simulink subsystem "Torque_vectoring_old"  (R2022a)
settings: Solver=VariableStepAuto  StartTime=0.0  StopTime=10.0  RelTol=1e-3
undefined symbols (not defined in the file): pac, param_vdc
libraries: slpidlib x1
settings Model: Creator=jutri  LastModifiedBy=Usuario
settings ModelReferenceCC: EnableRefExpFcnMdlSchedulingChecks=off
settings RTWCC: Description=Generic Real-Time Target  GPUComputeCapability=5.0

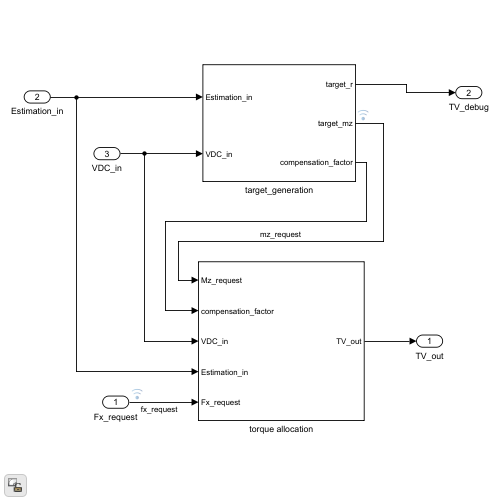
[thumbnail: Simulink's stored preview of the top-level diagram]
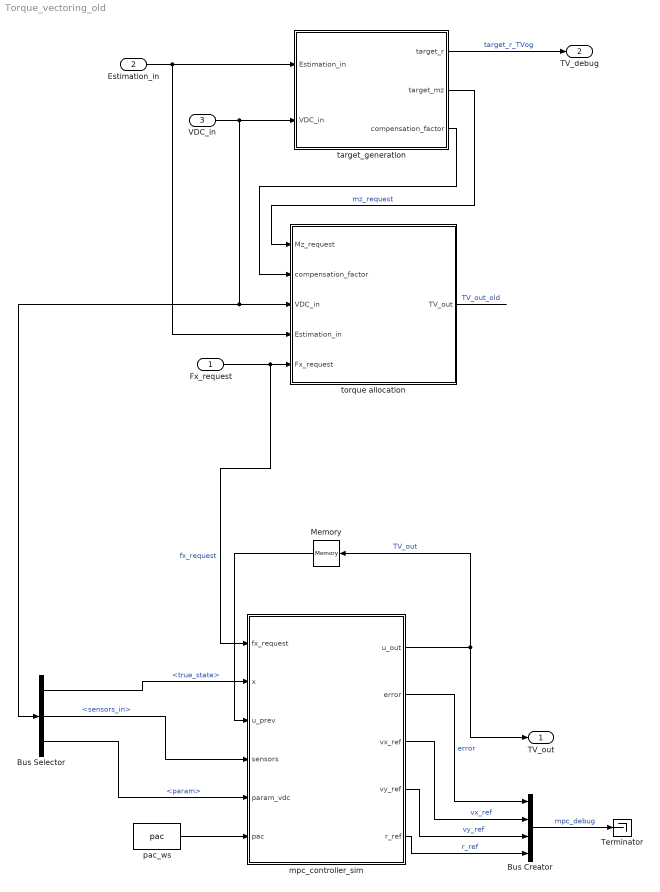
== system Torque_vectoring_old ==
  Fx_request : Inport
  Estimation_in : Inport  Port=2
  VDC_in : Inport  Port=3
  Bus Creator : BusCreator  Inputs=4
  Bus Selector : BusSelector  OutputSignals=true_state,sensors_in,param
  Memory : Memory  InitialCondition=[0;0;0;0]
  Terminator : Terminator
  mpc_controller_sim : MATLAB Function  TreatAsAtomicUnit=on
  pac_ws : Constant  Value=pac  OutDataTypeStr=Bus: pacBus
  target_generation : Subsystem
  torque allocation : Subsystem
  TV_out : Outport
  TV_debug : Outport  Port=2
  wires:
  Fx_request/1 -> torque allocation/5(Fx_request), mpc_controller_sim/1(fx_request)  "fx_request"
  torque allocation/1(TV_out) -> ?  "TV_out_old"
  target_generation/1(target_r) -> TV_debug/1  "target_r_TVog"
  Estimation_in/1 -> torque allocation/4(Estimation_in), target_generation/1(Estimation_in)
  VDC_in/1 -> Bus Selector/1, torque allocation/3(VDC_in), target_generation/2(VDC_in)
  target_generation/2(target_mz) -> torque allocation/1(Mz_request)  "mz_request"
  target_generation/3(compensation_factor) -> torque allocation/2(compensation_factor)
  mpc_controller_sim/1(u_out) -> Memory/1, TV_out/1  "TV_out"
  Memory/1 -> mpc_controller_sim/3(u_prev)
  Bus Selector/3 -> mpc_controller_sim/5(param_vdc)  "<param>"
  Bus Selector/2 -> mpc_controller_sim/4(sensors)  "<sensors_in>"
  Bus Selector/1 -> mpc_controller_sim/2(x)  "<true_state>"
  pac_ws/1 -> mpc_controller_sim/6(pac)
  mpc_controller_sim/2(error) -> Bus Creator/1  "error"
  Bus Creator/1 -> Terminator/1  "mpc_debug"
  mpc_controller_sim/3(vx_ref) -> Bus Creator/2  "vx_ref"
  mpc_controller_sim/4(vy_ref) -> Bus Creator/3  "vy_ref"
  mpc_controller_sim/5(r_ref) -> Bus Creator/4  "r_ref"

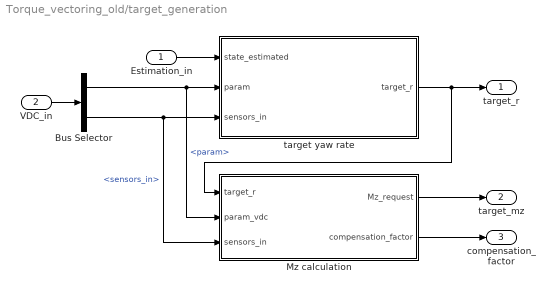
== system Torque_vectoring_old/target_generation ==
  Estimation_in : Inport
  VDC_in : Inport  Port=2
  Bus Selector : BusSelector  OutputSignals=param,sensors_in
  Mz calculation : Subsystem
  target yaw rate : Subsystem
  target_r : Outport
  target_mz : Outport  Port=2
  compensation_factor : Outport  Port=3
  wires:
  Mz calculation/2(compensation_factor) -> compensation_factor/1
  Bus Selector/2 -> target yaw rate/3(sensors_in), Mz calculation/3(sensors_in)  "<sensors_in>"
  Bus Selector/1 -> target yaw rate/2(param), Mz calculation/2(param_vdc)  "<param>"
  Estimation_in/1 -> target yaw rate/1(state_estimated)
  target yaw rate/1(target_r) -> target_r/1, Mz calculation/1(target_r)
  Mz calculation/1(Mz_request) -> target_mz/1
  VDC_in/1 -> Bus Selector/1

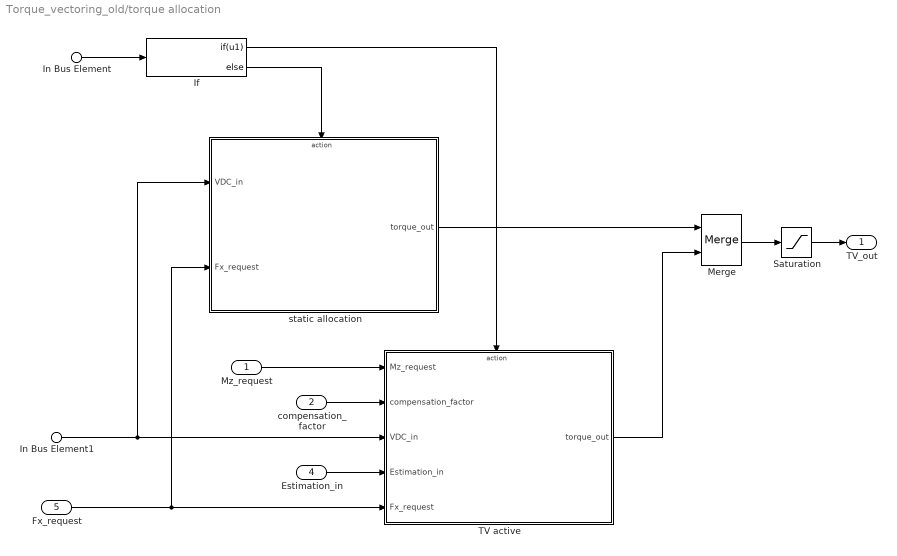
== system Torque_vectoring_old/torque allocation ==
  Mz_request : Inport
  compensation_factor : Inport  Port=2
  In Bus Element1 : Inport  Port=3  PortName=VDC_in
  In Bus Element : Inport  Port=3  PortName=VDC_in  Element=param.TV_active
  Estimation_in : Inport  Port=4
  Fx_request : Inport  Port=5
  If : If  IfExpression=u1
  Merge : Merge
  Saturation : Saturate  UpperLimit=param_vdc.torque_limit_positive  LowerLimit=param_vdc.torque_limit_negative
  TV active : Subsystem  TreatAsAtomicUnit=on
  static allocation : Subsystem  TreatAsAtomicUnit=on
  TV_out : Outport
  wires:
  compensation_factor/1 -> TV active/2(compensation_factor)
  Saturation/1 -> TV_out/1
  In Bus Element/1 -> If/1
  If/2 -> static allocation/Action
  If/1 -> TV active/Action
  Merge/1 -> Saturation/1
  TV active/1(torque_out) -> Merge/2
  static allocation/1(torque_out) -> Merge/1
  In Bus Element1/1 -> TV active/3(VDC_in), static allocation/1(VDC_in)
  Fx_request/1 -> TV active/5(Fx_request), static allocation/2(Fx_request)
  Estimation_in/1 -> TV active/4(Estimation_in)
  Mz_request/1 -> TV active/1(Mz_request)

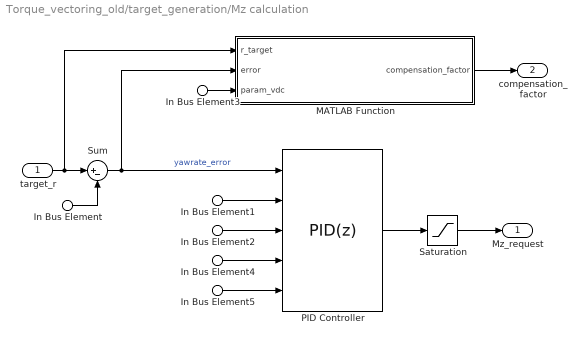
== system Torque_vectoring_old/target_generation/Mz calculation ==
  target_r : Inport
  In Bus Element3 : Inport  Port=2  PortName=param_vdc
  In Bus Element1 : Inport  Port=2  PortName=param_vdc  Element=TV_Kp
  In Bus Element2 : Inport  Port=2  PortName=param_vdc  Element=TV_Ki
  In Bus Element4 : Inport  Port=2  PortName=param_vdc  Element=TV_Kd
  In Bus Element5 : Inport  Port=2  PortName=param_vdc  Element=TV_N
  In Bus Element : Inport  Port=3  PortName=sensors_in  Element=IMU.r
  MATLAB Function : MATLAB Function  TreatAsAtomicUnit=on
  PID Controller : slpidlib/PID Controller  Controller=PID  Form=Parallel  TimeDomain=Discrete-time  UseExternalTs=off  SampleTime=-1  IntegratorMethod=Forward Euler  FilterMethod=Forward Euler  ControllerParametersSource=external  P=1  I=1  UseKiTs=off  D=0  N=100  UseFilter=on  TunerSelectOption=Transfer Function Based (PID Tuner App)  InitialConditionSource=internal  InitialConditionForIntegrator=0  InitialConditionForFilter=0  DifferentiatorICPrevScaledInput=0  ExternalReset=none  TrackingMode=off  Kt=1  LimitOutput=off  SatLimitsSource=internal  UpperSaturationLimit=inf  LowerSaturationLimit=-inf  LinearizeAsGain=on  AntiWindupMode=none  Kb=1  POutMin=[]  POutMax=[]  IOutMin=[]  IOutMax=[]  DOutMin=[]  DOutMax=[]  NOutMin=[]  NOutMax=[]  SumOutMin=[]  SumOutMax=[]  SaturationOutMin=[]  SaturationOutMax=[]  PParamMin=[]  PParamMax=[]  IParamMin=[]  IParamMax=[]  DParamMin=[]  DParamMax=[]  NParamMin=[]  NParamMax=[]  KbParamMin=[]  KbParamMax=[]  KtParamMin=[]  KtParamMax=[]  KbOutMin=[]  KbOutMax=[]  KtOutMin=[]  KtOutMax=[]  IntegratorOutMin=[]  IntegratorOutMax=[]  FilterOutMin=[]  FilterOutMax=[]  SumI1OutMin=[]  SumI1OutMax=[]  SumI2OutMin=[]  SumI2OutMax=[]  SumI3OutMin=[]  SumI3OutMax=[]  SumI4OutMin=[]  SumI4OutMax=[]  SumDOutMin=[]  SumDOutMax=[]  DifferentiatorOutMin=[]  DifferentiatorOutMax=[]  FilterDiffOutCoefMin=[]  FilterDiffOutCoefMax=[]  ReciprocalOutMin=[]  ReciprocalOutMax=[]  SumDenOutMin=[]  SumDenOutMax=[]  SumNumOutMin=[]  SumNumOutMax=[]  DivideOutMin=[]  DivideOutMax=[]  UdiffTsProdOutMin=[]  UdiffTsProdOutMax=[]  NTsProdOutMin=[]  NTsProdOutMax=[]  UintegralTsProdOutMin=[]  UintegralTsProdOutMax=[]  UngainTsProdOutMin=[]  UngainTsProdOutMax=[]  ClampingZeroOutDataTypeStr=Inherit: Inherit via back propagation  ClampingZeroOutMin=[]  ClampingZeroOutMax=[]  FilterDenConstantOutDataTypeStr=Inherit: Inherit via back propagation  FilterDenConstantOutMin=[]  FilterDenConstantOutMax=[]  PCopyOutDataTypeStr=Inherit: Inherit via back propagation  PCopyOutMin=[]  PCopyOutMax=[]  NCopyOutDataTypeStr=Inherit: Inherit via back propagation  NCopyOutMin=[]  NCopyOutMax=[]  IntegratorContinuousStateAttributes=''  IntegratorStateMustResolveToSignalObject=off  IntegratorRTWStateStorageClass=Auto  FilterContinuousStateAttributes=''  FilterStateMustResolveToSignalObject=off  FilterRTWStateStorageClass=Auto  ParallelPVariant=ExternalParameters  IdealPVariant=Disabled  IVariant=ExternalParameters  DVariant=ExternalParameters  IntegratorVariant=Discrete  SatVariant=Disabled  AWVariant=Passthrough  PCopyVariant=Disabled  TRVariant=Disabled  FdbkBlocksVariant=Forward  IdealPFdbkVariant=Disabled  SatFdbkVariant=Disabled  DerivativeFilterVariant=ForwardEulerFilter  NVariant=ExternalParameters  NCopyVariant=Disabled  FilterICVariant=InternalICsFilter  IntegratorICVariant=InternalICs  ExternalResetVariant=Disabled  TRSumVariant=Passthrough  SumFdbkVariant=Disabled  SumVariant=Sum_PID  TsampFilterVariant=InternalTs  TsampNgainVariant=Passthrough  TsampIntegralVariant=Passthrough  ExternalSaturationOutDataTypeStr=Inherit: Same as second input  aMode=0
  Saturation : Saturate  UpperLimit=param_vdc.max_mz  LowerLimit=-param_vdc.max_mz
  Sum : Sum  Inputs=|+-
  Mz_request : Outport
  compensation_factor : Outport  Port=2
  wires:
  MATLAB Function/1(compensation_factor) -> compensation_factor/1
  In Bus Element5/1 -> PID Controller/5
  In Bus Element4/1 -> PID Controller/4
  In Bus Element2/1 -> PID Controller/3
  In Bus Element1/1 -> PID Controller/2
  In Bus Element3/1 -> MATLAB Function/3(param_vdc)
  Sum/1 -> PID Controller/1, MATLAB Function/2(error)  "yawrate_error"
  In Bus Element/1 -> Sum/2
  target_r/1 -> Sum/1, MATLAB Function/1(r_target)
  PID Controller/1 -> Saturation/1
  Saturation/1 -> Mz_request/1

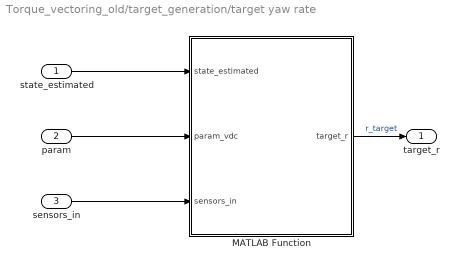
== system Torque_vectoring_old/target_generation/target yaw rate ==
  state_estimated : Inport
  param : Inport  Port=2
  sensors_in : Inport  Port=3
  MATLAB Function : MATLAB Function  TreatAsAtomicUnit=on
  target_r : Outport
  wires:
  MATLAB Function/1(target_r) -> target_r/1  "r_target"
  sensors_in/1 -> MATLAB Function/3(sensors_in)
  param/1 -> MATLAB Function/2(param_vdc)
  state_estimated/1 -> MATLAB Function/1(state_estimated)

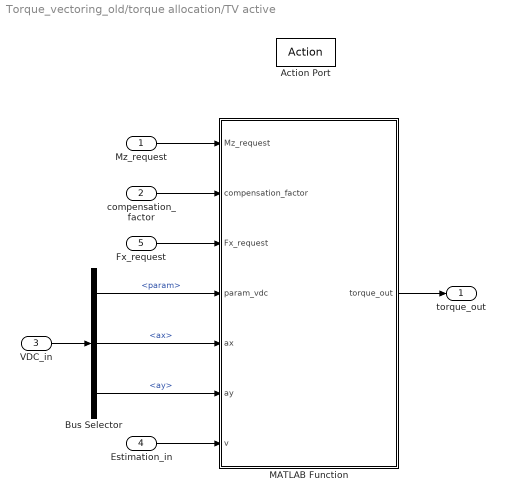
== system Torque_vectoring_old/torque allocation/TV active ==
  Mz_request : Inport
  compensation_factor : Inport  Port=2
  VDC_in : Inport  Port=3
  Estimation_in : Inport  Port=4
  Fx_request : Inport  Port=5
  Action Port : ActionPort
  Bus Selector : BusSelector  OutputSignals=param,sensors_in.IMU.ax,sensors_in.IMU.ay
  MATLAB Function : MATLAB Function  TreatAsAtomicUnit=on
  torque_out : Outport
  wires:
  compensation_factor/1 -> MATLAB Function/2(compensation_factor)
  Estimation_in/1 -> MATLAB Function/7(v)
  Fx_request/1 -> MATLAB Function/3(Fx_request)
  Mz_request/1 -> MATLAB Function/1(Mz_request)
  VDC_in/1 -> Bus Selector/1
  Bus Selector/1 -> MATLAB Function/4(param_vdc)  "<param>"
  Bus Selector/2 -> MATLAB Function/5(ax)  "<ax>"
  MATLAB Function/1(torque_out) -> torque_out/1
  Bus Selector/3 -> MATLAB Function/6(ay)  "<ay>"

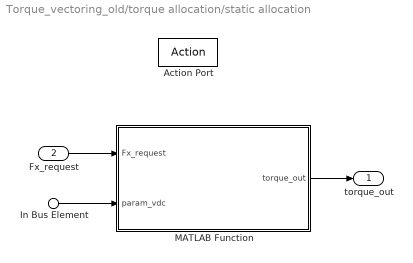
== system Torque_vectoring_old/torque allocation/static allocation ==
  In Bus Element : Inport  PortName=VDC_in  Element=param
  Fx_request : Inport  Port=2
  Action Port : ActionPort
  MATLAB Function : MATLAB Function  TreatAsAtomicUnit=on
  torque_out : Outport
  wires:
  Fx_request/1 -> MATLAB Function/1(Fx_request)
  In Bus Element/1 -> MATLAB Function/2(param_vdc)
  MATLAB Function/1(torque_out) -> torque_out/1

== matlab function Torque_vectoring_old/target_generation/target yaw rate/MATLAB Function ==
  data: state_estimated input; target_r output; param_vdc input; sensors_in input
function target_r = fcn(state_estimated, param_vdc, sensors_in)

delta = sensors_in.ext.steering;

% Kinematic bycicle model as ideal car
target_r = tan(delta) * state_estimated(1) / param_vdc.wheelbase;

== matlab function Torque_vectoring_old/torque allocation/TV active/MATLAB Function ==
  data: Mz_request input; compensation_factor input; torque_out output; Fx_request input; param_vdc input; ax input; ay input; v input
function torque_out = torque_allocation(Mz_request, compensation_factor, Fx_request, param_vdc, ax, ay, v)
% Input: Mz_request [Nm]
%        Fx_request [N]
%        ax         [m/s^2]
%        ay         [m/s^2]
%        v          [m/s]
%
% Output: 4x1 torque_out [Nm] (motor torque)
%
%     Se distribuye la comanda de par entre las cuatro ruedas respetando:
%       - sum(fx_tv) = Fx_request
%       - sum(mz asociado a cada rueda) = Mz_request
%       - reparto longitudinal proporcional a lambda_fx
%       - reparto de Mz proporcional a lambda_mz
%     donde sum(lambda_fx) = 1, sum(abs(lambda_mz))=1, sum(lambda_mz)=0


%% 2WD torque vectoring 
% torque_out = zeros(4,1);
% torque_out(3) = param_vdc.rdyn/param_vdc.gear_ratio*(0.5*Fx_request-Mz_request/param_vdc.trackwidthR);
% torque_out(4) = param_vdc.rdyn/param_vdc.gear_ratio*(0.5*Fx_request+Mz_request/param_vdc.trackwidthR);

%% 4WD torque vectoring

if param_vdc.TV_use_fz
    tire_loads = calculate_tire_loads_vdc(ax,ay,v(1),param_vdc);
    fz_front_mean = mean(tire_loads(1:2));
    fz_rear_mean = mean(tire_loads(3:4));

    lambda_fx = [fz_front_mean; fz_front_mean; fz_rear_mean; fz_rear_mean] / sum(tire_loads);
    lambda_mz = tire_loads ./ sum(tire_loads) .* [-1;1;-1;1];
else
    dist_f = param_vdc.TV_front;
    dist_r = param_vdc.TV_rear;

    lambda_fx = 0.5 * [dist_f; dist_f; dist_r; dist_r];
    lambda_mz = 0.5 * [-dist_f; dist_f; -dist_r; dist_r];
end

% Compensation factor para sub/sobreviraje
if param_vdc.TV_use_compensation
    lambda_fx = lambda_fx + compensation_factor * [-1; -1; 1; 1];
    lambda_mz = lambda_mz + compensation_factor * [-1; -1; 1; 1];
end

% Calculamos el reparto según los coeficientes
fx_tv = lambda_fx * Fx_request + lambda_mz * 2 * Mz_request / param_vdc.trackwidthF; % track front y rear son iguales
torque_out = param_vdc.rdyn * fx_tv / param_vdc.gear_ratio;

% Compensamos saturación de alguna rueda para alcanzar fx_request
real_torque = max(param_vdc.torque_limit_negative,min(param_vdc.torque_limit_positive, torque_out));
free_mot = torque_out <= real_torque;
real_fx = sum(real_torque);

torque_out = torque_out + param_vdc.rdyn/param_vdc.gear_ratio*(Fx_request - real_fx).*free_mot / sum(free_mot);

== matlab function Torque_vectoring_old/torque allocation/static allocation/MATLAB Function ==
  data: torque_out output; Fx_request input; param_vdc input
function torque_out = fcn(Fx_request, param_vdc)

% Output: 4x1 torque_out [Nm] (motor torque)
torque_out = param_vdc.rdyn / param_vdc.gear_ratio * Fx_request * param_vdc.static_torque_distribution;

== matlab function Torque_vectoring_old/target_generation/Mz calculation/MATLAB Function ==
  data: r_target input; compensation_factor output; error input; param_vdc input
function compensation_factor = understeer_compensation(r_target, error, param_vdc)

if ((r_target > 0) && (error < 0)) || ((r_target < 0) && (error > 0))
    % Oversteer
    compensation_factor = - param_vdc.max_compensation * abs(error) / param_vdc.max_yawrate_error;
    compensation_factor = max(compensation_factor, -param_vdc.max_compensation);
else
    % Understeer
    compensation_factor = param_vdc.max_compensation * abs(error) / param_vdc.max_yawrate_error;
    compensation_factor = min(compensation_factor, param_vdc.max_compensation);
end

== matlab function Torque_vectoring_old/mpc_controller_sim ==
  data: fx_request input; x input; u_out output; u_prev input; sensors input; param_vdc input; pac input; error output; vx_ref output; vy_ref output; r_ref output
function [u_out, error, vx_ref, vy_ref, r_ref] = mpc_controller_sim(fx_request, x, u_prev, sensors, param_vdc, pac)
    [u_out, error, vx_ref, vy_ref, r_ref] = mpc_controller(fx_request, x, u_prev, sensors, param_vdc, pac);
end
